simulink library "ddm"  (R2021b)
settings: Solver=VariableStepAuto  StartTime=0.0  StopTime=10.0  RelTol=1e-3
undefined symbols (not defined in the file or in its folder): ENUM_ADASACCSTA_ERROR, ENUM_ADASACCSTA_OFF, ENUM_ADASACCSTA_STANDBY, ENUM_ADASISASTA_OFF, ENUM_ALLOWMOV_ALLOWREADY, ENUM_APS, ENUM_BRKSTA_ERROR, ENUM_BRKSTA_OFF, ENUM_BRKSTA_ON, ENUM_CHGPREACTERRSTA_OBCPRE, ENUM_DCDCFAULTSTA_ANYFAULTLV1, ENUM_DCDCFAULTSTA_ANYFAULTLV2, ENUM_DRIVETRAIN_AWD, ENUM_DRIVETRAIN_FWD, ENUM_DRIVETRAIN_RWD, ENUM_DRSEATSTA_INVALID, ENUM_EDUDRTSTA_NORMAL, ENUM_EPBSTA_APPLIED, ENUM_EPBSTA_RELEASED, ENUM_HVBATTREADYPRE_READY, ENUM_MCUWARN_LV0, ENUM_MCUWARN_LV1, ENUM_MCUWARN_LV2, ENUM_MCUWARN_LV3, ENUM_MCUWARN_NOERROR, ENUM_OBCFAULTSTA_ANYFAULT, ENUM_PAS_R2F2, ENUM_PDFAULT_BATTPDFAIL, ENUM_PDFAULT_DCDCDISABLE, ENUM_PDFAULT_MCUDISABLE, ENUM_PDFAULT_MCUDISCHRG, ENUM_POWERSTA_OFF, ENUM_POWERSTA_ON, ENUM_POWERSTA_READY, ENUM_POWERSTA_STANDBY, ENUM_PRESSINDI_LOW, ENUM_PUFAULT_BATTUPFAIL, ENUM_PUFAULT_DCDCENABLEFAIL, ENUM_PUFAULT_PRECHRGCHKFAIL, ENUM_PUFAULT_SAFETYCHKFAIL, ENUM_PUSTATE_COMPLETED, ENUM_PWRSTASW_OFF, ENUM_PWRSTASW_OFFA, ENUM_PWRSTASW_OFFCHVCHRG, ENUM_PWRSTASW_OFFCLVCHRG, ENUM_PWRSTASW_ON, ENUM_PWRSTASW_ONHVCHRG, ENUM_PWRSTASW_READY, ENUM_PWRSTASW_STANDBY, ENUM_RANGESTA_12IN, ENUM_RANGESTA_12OUT, ENUM_SHIFTCOMMAND_D, ENUM_SHIFTCOMMAND_N, ENUM_SHIFTCOMMAND_P, ENUM_SHIFTCOMMAND_R, ENUM_ZONEMALFUNLV_1ST, ENUM_ZONEMALFUNLV_2ND, ENUM_ZONEMALFUNLV_3RD, ENUM_ZONEMALFUNLV_4TH, ENUM_ZONESPDCTRLMODE_ACC ... (+832)
libraries: hcu_lib x738, $bdroot x26, simulink x7
(part 15 of 25)

== system ddm/DDM/DDM/PMM/Comm err/VCU lost communication with CCU1 ==
  note: Fail Safe During Detection
  note: Test Pass Criteria
  note: Test Detection Criteria
  note: Fail Safe After Decision
  note: Release Condition After Failure Decision
  note: Release Condition During Failure Detection
  task_time_s : Inport
  VPMM_PowerSta_enum : Inport  Port=2
  VPMM_PwrStaSW_enum : Inport  Port=3
  VDDM_C3CCU1LCChk_flg : Inport  Port=4
  No_CAN3_BUS_OFF : Inport  Port=5
  DTC_clear_request : Inport  Port=6
  Constant15 : Constant  Value=KDDM_C3CCU1LCCFSSW_flg
  Constant{3,16,22,24} (4 alike) : Constant  Value=TRUE
  Constant18 : Constant  Value=KDDM_C3CCU1LCPassTO_s
  Constant19 : Constant  Value=KDDM_C3CCU1LCPassTO_s
  Constant{2,21,23,25,27} (5 alike) : Constant  Value=FALSE
  Constant20 : Constant  Value=KDDM_C3CCU1LCDFSSW_flg
  Constant26 : Constant  Value=ENUM_PWRSTASW_OFF
  Constant28 : Constant  Value=ENUM_PWRSTASW_OFF
  Constant4 : Constant  Value=ENUM_POWERSTA_OFF
  Constant40 : Constant  Value=KDDM_C3CCU1LCDTC_cnt
  Constant41 : Constant  Value=KDDM_C3CCU1LCDetTO_s
  Constant46 : Constant  Value=KDDM_C3CCU1LCDetSW_flg
  Constant48 : Constant  Value=KDDM_C3CCU1LCDTC_cnt
  Constant5 : Constant  Value=KDDM_C3CCU1LCPassSW_flg
  DTC_Couter : hcu_lib/Basic_Blocks/DTC_Couter
  DTC_Info : hcu_lib/Basic_Blocks/DTC_Info
  Data Type Conversion1 : DataTypeConversion  OutDataTypeStr=uint8
  Demux : Demux  Commented=on  Outputs=5
  Equal : RelationalOperator  Operator=~=  OutDataTypeStr=boolean  RndMeth=Simplest
  Equal2 : RelationalOperator  Operator=~=  OutDataTypeStr=boolean  RndMeth=Simplest
  Equal3 : RelationalOperator  OutDataTypeStr=boolean  RndMeth=Simplest
  Equal4 : RelationalOperator  Operator===  OutDataTypeStr=boolean  RndMeth=Simplest
  From19 : From  Commented=on  GotoTag=VDDM_C3CCU1LCDFS_flg
  Goto19 : Goto  Commented=on  GotoTag=VDDM_EDriveSysErrVCUErr_flg
  Logical Operator{2,5,12,15,18..19} (6 alike) : Logic  AllPortsSameDT=off  OutDataTypeStr=boolean
  Logical Operator21 : Logic  Operator=OR  AllPortsSameDT=off  OutDataTypeStr=boolean
  Logical Operator3 : Logic  Operator=OR  AllPortsSameDT=off  OutDataTypeStr=boolean
  Logical Operator6 : Logic  Operator=NOT  AllPortsSameDT=off  OutDataTypeStr=boolean
  Logical Operator8 : Logic  Operator=OR  AllPortsSameDT=off  OutDataTypeStr=boolean
  Relay : Relay  OnSwitchValue=ONE_INT  OffSwitchValue=ZERO_INT
  SR_Latch1 : Subsystem  mask(SR_Latch){}
      mask help: SR latch function.
  SR_Latch3 : hcu_lib/Basic_Blocks/SR_Latch
  SR_Latch4 : hcu_lib/Basic_Blocks/SR_Latch
  Switch{,1,4..7} (6 alike) : Switch  Criteria=u2 ~= 0
  Switch3 : Switch  Commented=on  Criteria=u2 ~= 0
  Test Detection Criteria : hcu_lib/Basic_Blocks/Test Detection Criteria
  Timer1 : hcu_lib/Basic_Blocks/Timer
  Unit Delay3 : UnitDelay  Commented=on  SampleTime=-1  HasFrameUpgradeWarning=on
  VDDM_C3CCU1LCDTC_raw32 : Outport
  VDDM_C3CCU1LCCFS_flg : Outport  Port=2
  wires:
  VPMM_PowerSta_enum/1 -> [VPMM_PowerSta_enum]
  VPMM_PwrStaSW_enum/1 -> [VPMM_PwrStaSW_enum]
  VDDM_C3CCU1LCChk_flg/1 -> [VDDM_C3CCU1LCChk_flg]
  task_time_s/1 -> [task_time_s]
  DTC_clear_request/1 -> [DTC_clear_request]
  No_CAN3_BUS_OFF/1 -> [No_CAN3_BUS_OFF]
  Equal4/1 -> Logical Operator8/1
  Switch4/1 -> [VDDM_C3CCU1LCCFSRls_flg]
  Constant20/1 -> Logical Operator12/1
  Constant25/1 -> Switch4/3
  [DTC_clear_request] -> Logical Operator8/2
  [VDDM_C3CCU1LCChk_flg] -> Switch6/1
  Equal3/1 -> SR_Latch1/1(set)
  Logical Operator8/1 -> Switch4/2
  SR_Latch1/1(latched) -> [VDDM_C3CCU1LCPass_flg]
  Switch7/1 -> [VDDM_C3CCU1LCDFSRls_flg]
  Constant46/1 -> Logical Operator19/2
  [VDDM_C3CCU1LCChk_flg] -> Switch5/1
  Constant23/1 -> Switch7/3
  From19/1 -> Switch3/2
  Test Detection Criteria/1 -> [VDDM_C3CCU1LCDet_flg]  "VDDM_C3CCU1LCDet_flg"
  Constant27/1 -> Switch5/3
  Switch6/1 -> Logical Operator6/1, Timer1/2
  Timer1/1 -> Equal3/1
  Constant16/1 -> Switch6/3
  Constant18/1 -> Timer1/4
  [VDDM_C3CCU1LCCFS_flg] -> Logical Operator21/2
  Equal2/1 -> Logical Operator5/2
  Switch/1 -> Goto19/1
  Constant26/1 -> Equal/2
  [VDDM_xxx_flg] -> SR_Latch1/2(reset)
  Data Type Conversion1/1 -> [VDDM_C3CCU1LCDTC_cnt]  "VDDM_C3CCU1LCDTC_cnt"
  Constant40/1 -> Test Detection Criteria/3
  [VDDM_C3CCU1LCCFSRls_flg] -> SR_Latch4/2
  DTC_Couter/1 -> SR_Latch4/1
  [No_CAN3_BUS_OFF] -> Logical Operator5/1
  Logical Operator18/1 -> [VDDM_C3CCU1LCCFS_flg]
  Logical Operator3/1 -> Logical Operator15/1
  [VDDM_C3CCU1LCPass_flg] -> Switch7/2
  Constant5/1 -> Logical Operator15/2
  Logical Operator2/1 -> Switch5/2
  Constant15/1 -> Logical Operator18/2
  Constant48/1 -> DTC_Couter/3
  Constant28/1 -> Equal2/2
  [VDDM_C3CCU1LCCFSRls_flg] -> Logical Operator3/2
  [VDDM_C3CCU1LCCFS_flg] -> Switch/2
  [No_CAN3_BUS_OFF] -> Logical Operator2/1
  [VDDM_C3CCU1LCPass_flg] -> Logical Operator3/1
  Logical Operator12/1 -> [VDDM_C3CCU1LCDFS_flg]
  Logical Operator21/1 -> SR_Latch3/2
  DTC_Couter/2 -> Data Type Conversion1/1
  Constant22/1 -> Switch7/1
  SR_Latch3/1 -> Logical Operator12/2
  Constant3/1 -> Switch/1
  Constant21/1 -> Switch/3
  Switch3/1 -> Demux/1
  [VDDM_C3CCU1LCDTC_cnt] -> Relay/1
  SR_Latch4/1 -> Logical Operator18/1
  Logical Operator5/1 -> Switch6/2
  Relay/1 -> SR_Latch3/1
  [VDDM_C3CCU1LCDFSRls_flg] -> Logical Operator21/1
  Constant4/1 -> Equal4/2
  [VDDM_C3CCU1LCDet_flg] -> Logical Operator19/1
  Logical Operator19/1 -> DTC_Couter/1
  Constant19/1 -> Equal3/2
  Logical Operator6/1 -> Timer1/1
  Equal/1 -> Logical Operator2/2
  [task_time_s] -> Test Detection Criteria/2
  Logical Operator15/1 -> DTC_Couter/2
  Demux/1 -> Unit Delay3/1
  Constant24/1 -> Switch4/1
  [VPMM_PowerSta_enum] -> Equal4/1
  [VPMM_PwrStaSW_enum] -> Equal/1
  [VPMM_PwrStaSW_enum] -> Equal2/1
  [task_time_s] -> Timer1/3
  DTC_Info/1 -> VDDM_C3CCU1LCDTC_raw32/1  "VDDM_C3CCU1LCDTC_raw32"
  [VDDM_C3CCU1LCPass_flg] -> DTC_Info/2
  [VDDM_C3CCU1LCCFS_flg] -> DTC_Info/3, VDDM_C3CCU1LCCFS_flg/1
  [VDDM_C3CCU1LCDet_flg] -> DTC_Info/1
  Constant41/1 -> Test Detection Criteria/4
  [DTC_clear_request] -> DTC_Info/4
  [DTC_clear_request] -> Switch1/2
  Switch1/1 -> Test Detection Criteria/1
  Switch5/1 -> [VDDM_xxx_flg], Switch1/3
  Constant2/1 -> Switch1/1

== system ddm/DDM/DDM/PMM/Comm err/VCU lost communication with CCU2 ==
  note: Fail Safe After Decision
  note: Test Pass Criteria
  note: Release Condition After Failure Decision
  note: Fail Safe During Detection
  note: Release Condition During Failure Detection
  note: Diagnostics and Fault Handling
  note: Test Detection Criteria
  task_time_s : Inport
  VPMM_PowerSta_enum : Inport  Port=2
  VPMM_PwrStaSW_enum : Inport  Port=3
  VDDM_C3CCU2LCChk_flg : Inport  Port=4
  No_CAN3_BUS_OFF : Inport  Port=5
  DTC_clear_request : Inport  Port=6
  Constant15 : Constant  Value=KDDM_C3CCU2LCCFSSW_flg
  Constant{3,16,22,24} (4 alike) : Constant  Value=TRUE
  Constant18 : Constant  Value=KDDM_C3CCU2LCPassTO_s
  Constant19 : Constant  Value=KDDM_C3CCU2LCPassTO_s
  Constant{2,21,23,25,27} (5 alike) : Constant  Value=FALSE
  Constant20 : Constant  Value=KDDM_C3CCU2LCDFSSW_flg
  Constant26 : Constant  Value=ENUM_PWRSTASW_OFF
  Constant28 : Constant  Value=ENUM_PWRSTASW_OFF
  Constant4 : Constant  Value=ENUM_POWERSTA_OFF
  Constant40 : Constant  Value=KDDM_C3CCU2LCDTC_cnt
  Constant41 : Constant  Value=KDDM_C3CCU2LCDetTO_s
  Constant46 : Constant  Value=KDDM_C3CCU2LCDetSW_flg
  Constant48 : Constant  Value=KDDM_C3CCU2LCDTC_cnt
  Constant5 : Constant  Value=KDDM_C3CCU2LCPassSW_flg
  DTC_Couter : hcu_lib/Basic_Blocks/DTC_Couter
  DTC_Info : hcu_lib/Basic_Blocks/DTC_Info
  Data Type Conversion1 : DataTypeConversion  OutDataTypeStr=uint8
  Demux : Demux  Commented=on  Outputs=5
  Equal : RelationalOperator  Operator=~=  OutDataTypeStr=boolean  RndMeth=Simplest
  Equal2 : RelationalOperator  Operator=~=  OutDataTypeStr=boolean  RndMeth=Simplest
  Equal3 : RelationalOperator  OutDataTypeStr=boolean  RndMeth=Simplest
  Equal4 : RelationalOperator  Operator===  OutDataTypeStr=boolean  RndMeth=Simplest
  From19 : From  Commented=on  GotoTag=VDDM_C3CCU2LCDFS_flg
  Goto19 : Goto  Commented=on  GotoTag=VDDM_EDriveSysErrVCUErr_flg
  Logical Operator{2,5,12,15,18..19} (6 alike) : Logic  AllPortsSameDT=off  OutDataTypeStr=boolean
  Logical Operator21 : Logic  Operator=OR  AllPortsSameDT=off  OutDataTypeStr=boolean
  Logical Operator3 : Logic  Operator=OR  AllPortsSameDT=off  OutDataTypeStr=boolean
  Logical Operator6 : Logic  Operator=NOT  AllPortsSameDT=off  OutDataTypeStr=boolean
  Logical Operator8 : Logic  Operator=OR  AllPortsSameDT=off  OutDataTypeStr=boolean
  Relay : Relay  OnSwitchValue=ONE_INT  OffSwitchValue=ZERO_INT
  SR_Latch1 : Subsystem  mask(SR_Latch){}
      mask help: SR latch function.
  SR_Latch3 : hcu_lib/Basic_Blocks/SR_Latch
  SR_Latch4 : hcu_lib/Basic_Blocks/SR_Latch
  Switch{,1,4..7} (6 alike) : Switch  Criteria=u2 ~= 0
  Switch3 : Switch  Commented=on  Criteria=u2 ~= 0
  Test Detection Criteria : hcu_lib/Basic_Blocks/Test Detection Criteria
  Timer1 : hcu_lib/Basic_Blocks/Timer
  Unit Delay3 : UnitDelay  Commented=on  SampleTime=-1  HasFrameUpgradeWarning=on
  VDDM_C3CCU2LCDTC_raw32 : Outport
  VDDM_C3CCU2LCCFS_flg : Outport  Port=2
  wires:
  task_time_s/1 -> [task_time_s]
  VDDM_C3CCU2LCChk_flg/1 -> [VDDM_C3CCU2LCChk_flg]
  VPMM_PwrStaSW_enum/1 -> [VPMM_PwrStaSW_enum]
  VPMM_PowerSta_enum/1 -> [VPMM_PowerSta_enum]
  No_CAN3_BUS_OFF/1 -> [No_CAN3_BUS_OFF]
  DTC_clear_request/1 -> [DTC_clear_request]
  Switch/1 -> Goto19/1
  Constant26/1 -> Equal/2
  Equal2/1 -> Logical Operator5/2
  [VDDM_C3CCU2LCCFS_flg] -> Logical Operator21/2
  Constant40/1 -> Test Detection Criteria/3
  Data Type Conversion1/1 -> [VDDM_C3CCU2LCDTC_cnt]  "VDDM_C3CCU2LCDTC_cnt"
  [VDDM_xxx_flg] -> SR_Latch1/2(reset)
  Logical Operator18/1 -> [VDDM_C3CCU2LCCFS_flg]
  [No_CAN3_BUS_OFF] -> Logical Operator5/1
  DTC_Couter/1 -> SR_Latch4/1
  Constant46/1 -> Logical Operator19/2
  SR_Latch1/1(latched) -> [VDDM_C3CCU2LCPass_flg]
  Constant23/1 -> Switch7/3
  Switch7/1 -> [VDDM_C3CCU2LCDFSRls_flg]
  Logical Operator8/1 -> Switch4/2
  Equal3/1 -> SR_Latch1/1(set)
  [VDDM_C3CCU2LCChk_flg] -> Switch6/1
  Constant20/1 -> Logical Operator12/1
  [DTC_clear_request] -> Logical Operator8/2
  Constant25/1 -> Switch4/3
  Equal4/1 -> Logical Operator8/1
  Switch4/1 -> [VDDM_C3CCU2LCCFSRls_flg]
  Constant3/1 -> Switch/1
  Constant22/1 -> Switch7/1
  [VDDM_C3CCU2LCChk_flg] -> Switch5/1
  DTC_Couter/2 -> Data Type Conversion1/1
  Constant48/1 -> DTC_Couter/3
  [VDDM_C3CCU2LCCFSRls_flg] -> Logical Operator3/2
  Logical Operator12/1 -> [VDDM_C3CCU2LCDFS_flg]
  Constant15/1 -> Logical Operator18/2
  Constant28/1 -> Equal2/2
  [VDDM_C3CCU2LCCFS_flg] -> Switch/2
  Equal/1 -> Logical Operator2/2
  Logical Operator6/1 -> Timer1/1
  Constant24/1 -> Switch4/1
  Constant19/1 -> Equal3/2
  [task_time_s] -> Test Detection Criteria/2
  [No_CAN3_BUS_OFF] -> Logical Operator2/1
  [VDDM_C3CCU2LCPass_flg] -> Logical Operator3/1
  Constant4/1 -> Equal4/2
  [VDDM_C3CCU2LCDFSRls_flg] -> Logical Operator21/1
  Relay/1 -> SR_Latch3/1
  Constant21/1 -> Switch/3
  [VDDM_C3CCU2LCDet_flg] -> Logical Operator19/1
  SR_Latch4/1 -> Logical Operator18/1
  Logical Operator21/1 -> SR_Latch3/2
  [VDDM_C3CCU2LCDTC_cnt] -> Relay/1
  Demux/1 -> Unit Delay3/1
  Switch3/1 -> Demux/1
  Logical Operator19/1 -> DTC_Couter/1
  Test Detection Criteria/1 -> [VDDM_C3CCU2LCDet_flg]  "VDDM_C3CCU2LCDet_flg"
  From19/1 -> Switch3/2
  Constant18/1 -> Timer1/4
  Constant16/1 -> Switch6/3
  [VDDM_C3CCU2LCCFSRls_flg] -> SR_Latch4/2
  Timer1/1 -> Equal3/1
  Switch6/1 -> Logical Operator6/1, Timer1/2
  Constant27/1 -> Switch5/3
  Logical Operator5/1 -> Switch6/2
  Constant5/1 -> Logical Operator15/2
  SR_Latch3/1 -> Logical Operator12/2
  [VDDM_C3CCU2LCPass_flg] -> Switch7/2
  Logical Operator3/1 -> Logical Operator15/1
  Logical Operator15/1 -> DTC_Couter/2
  Logical Operator2/1 -> Switch5/2
  [VPMM_PowerSta_enum] -> Equal4/1
  [VPMM_PwrStaSW_enum] -> Equal/1
  [VPMM_PwrStaSW_enum] -> Equal2/1
  [task_time_s] -> Timer1/3
  DTC_Info/1 -> VDDM_C3CCU2LCDTC_raw32/1  "VDDM_C3CCU2LCDTC_raw32"
  [VDDM_C3CCU2LCPass_flg] -> DTC_Info/2
  [VDDM_C3CCU2LCCFS_flg] -> DTC_Info/3, VDDM_C3CCU2LCCFS_flg/1
  [VDDM_C3CCU2LCDet_flg] -> DTC_Info/1
  Constant41/1 -> Test Detection Criteria/4
  [DTC_clear_request] -> DTC_Info/4
  [DTC_clear_request] -> Switch1/2
  Switch1/1 -> Test Detection Criteria/1
  Switch5/1 -> [VDDM_xxx_flg], Switch1/3
  Constant2/1 -> Switch1/1

== system ddm/DDM/DDM/PMM/Fault level/Fault level 1 subsystem error ==
  note: Fail Safe Operation During Failure Detection
  note: Release Condition During Failure Detection
  note: Fail Safe Operation After Failure Decision
  note: Test Pass Criteria
  note: Test Detection Criteria
  note: Diagnostics and Fault Handling
  note: Release Condition After Failure Decision
  task_time_s : Inport
  VPMM_PowerSta_enum : Inport  Port=2
  VPMM_PwrStaSW_enum : Inport  Port=3
  VDDM_C3BMS6LCCFS_flg : Inport  Port=4
  VDDM_C3CCU2LCCFS_flg : Inport  Port=5
  VDDM_MCUF1NoComCFS_flg : Inport  Port=6
  VDDM_MCUR1NoComCFS_flg : Inport  Port=7
  VINP_BMSWarn1_flg : Inport  Port=8
  VINP_BMSWarn2_flg : Inport  Port=9
  VINP_BMSWarn3_flg : Inport  Port=10
  VINP_DCDCFaultSta_enum : Inport  Port=11
  VINP_MCUWarnF_enum : Inport  Port=12
  VINP_MCUWarnR_enum : Inport  Port=13
  VINP_OBCFaultSta_enum : Inport  Port=14
  VPMM_DrivetrainSelect_enum : Inport  Port=15
  DTC_clear_request : Inport  Port=16
  No_CAN3_BUS_OFF : Inport  Port=17
  Constant : Constant  Value=KDDM_Lv1ErrDetTO_s
  Constant1 : Constant  Value=KDDM_Lv1ErrPassTO_s
  Constant{5,10,42,47} (4 alike) : Constant  Value=ENUM_MCUWARN_LV0
  Constant{6,11,43,49} (4 alike) : Constant  Value=ENUM_DRIVETRAIN_AWD
  Constant12 : Constant  Value=KDDM_Lv1ErrDTC_cnt
  Constant13 : Constant  Value=KDDM_Lv1ErrDetSW_flg
  Constant14 : Constant  Value=KDDM_Lv1ErrPassSW_flg
  Constant{15,21,25,27} (4 alike) : Constant  Value=FALSE
  Constant18 : Constant  Value=KDDM_Lv1ErrPassTO_s
  Constant2 : Constant  Value=KDDM_Lv1ErrCFSSW_flg
  Constant24 : Constant  Value=TRUE
  Constant26 : Constant  Value=ENUM_PWRSTASW_OFF
  Constant3 : Constant  Value=TRUE
  Constant36 : Constant  Value=ENUM_DCDCFAULTSTA_ANYFAULTLV1
  Constant37 : Constant  Value=ENUM_OBCFAULTSTA_ANYFAULT
  Constant38 : Constant  Value=ENUM_PWRSTASW_OFF
  Constant39 : Constant  Value=TRUE
  Constant4 : Constant  Value=ENUM_POWERSTA_OFF
  Constant40 : Constant  Value=KDDM_Lv1ErrDTC_cnt
  Constant44 : Constant  Value=ENUM_DRIVETRAIN_FWD
  Constant45 : Constant  Value=ENUM_DRIVETRAIN_RWD
  Constant50 : Constant  Value=ENUM_DCDCFAULTSTA_ANYFAULTLV1
  Constant51 : Constant  Value=ENUM_OBCFAULTSTA_ANYFAULT
  Constant7 : Constant  Value=ENUM_DRIVETRAIN_FWD
  Constant8 : Constant  Value=ENUM_DRIVETRAIN_RWD
  Constant9 : Constant  Value=KDDM_Lv1ErrDFSSW_flg
  DTC_Couter : hcu_lib/Basic_Blocks/DTC_Couter
  DTC_Info : hcu_lib/Basic_Blocks/DTC_Info
  Data Type Conversion1 : DataTypeConversion  OutDataTypeStr=uint8
  Equal : RelationalOperator  Operator=~=  OutDataTypeStr=boolean  RndMeth=Simplest
  Equal{1,4..9,14..21,25..26} (17 alike) : RelationalOperator  Operator===  OutDataTypeStr=boolean  RndMeth=Simplest
  Equal2 : RelationalOperator  Operator=~=  OutDataTypeStr=boolean  RndMeth=Simplest
  Equal3 : RelationalOperator  OutDataTypeStr=boolean  RndMeth=Simplest
  Goto24 : Goto  Commented=on  GotoTag=VDDM_EDriveSysErrVCUErr_flg
  Logical Operator{1,4..7,9..10,27..28} (9 alike) : Logic  Operator=NOT  AllPortsSameDT=off  OutDataTypeStr=boolean
  Logical Operator11 : Logic  Operator=OR  Inputs=7  AllPortsSameDT=off  OutDataTypeStr=boolean
  Logical Operator{12..13,15..16,18..19,22,24} (8 alike) : Logic  AllPortsSameDT=off  OutDataTypeStr=boolean
  Logical Operator{3,8,14,17,23,25} (6 alike) : Logic  Operator=OR  AllPortsSameDT=off  OutDataTypeStr=boolean
  Logical Operator2 : Logic  Inputs=6  AllPortsSameDT=off  OutDataTypeStr=boolean
  Logical Operator20 : Logic  Operator=OR  Inputs=7  AllPortsSameDT=off  OutDataTypeStr=boolean
  Logical Operator26 : Logic  Inputs=6  AllPortsSameDT=off  OutDataTypeStr=boolean
  Relay : Relay  OnSwitchValue=ONE_INT  OffSwitchValue=ZERO_INT
  SR_Latch1 : Subsystem  mask(SR_Latch){}
      mask help: SR latch function.
  SR_Latch3 : hcu_lib/Basic_Blocks/SR_Latch
  SR_Latch4 : hcu_lib/Basic_Blocks/SR_Latch
  Switch{,2,4..6} (5 alike) : Switch  Criteria=u2 ~= 0
  Test Detection Criteria : hcu_lib/Basic_Blocks/Test Detection Criteria
  Timer1 : hcu_lib/Basic_Blocks/Timer
  VDDM_Lv1ErrDTC_raw32 : Outport
  wires:
  task_time_s/1 -> [task_time_s]
  VPMM_PwrStaSW_enum/1 -> [VPMM_PwrStaSW_enum]
  VPMM_PowerSta_enum/1 -> [VPMM_PowerSta_enum]
  VDDM_C3CCU2LCCFS_flg/1 -> [VDDM_C3CCU2LCCFS_flg]
  VPMM_DrivetrainSelect_enum/1 -> [VPMM_DrivetrainSelect_enum]
  VINP_MCUWarnR_enum/1 -> [VINP_MCUWarnR_enum]
  VDDM_MCUR1NoComCFS_flg/1 -> [VDDM_MCUR1NoComCFS_flg]
  VDDM_MCUF1NoComCFS_flg/1 -> [VDDM_MCUF1NoComCFS_flg]
  VINP_BMSWarn1_flg/1 -> [VINP_BMSWarn1_flg]
  VINP_BMSWarn2_flg/1 -> [VINP_BMSWarn2_flg]
  VINP_BMSWarn3_flg/1 -> [VINP_BMSWarn3_flg]
  VINP_DCDCFaultSta_enum/1 -> [VINP_DCDCFaultSta_enum]
  VINP_MCUWarnF_enum/1 -> [VINP_MCUWarnF_enum]
  VINP_OBCFaultSta_enum/1 -> [VINP_OBCFaultSta_enum]
  VDDM_C3BMS6LCCFS_flg/1 -> [VDDM_C3BMS6LCCFS_flg]
  Equal4/1 -> Logical Operator8/1
  Constant1/1 -> Timer1/4
  Relay/1 -> SR_Latch3/1
  DTC_Couter/2 -> Data Type Conversion1/1
  Constant21/1 -> Switch/3
  Constant2/1 -> Logical Operator18/2
  Switch/1 -> Goto24/1
  [DTC_clear_request] -> Logical Operator8/2
  Constant3/1 -> Switch/1
  [VDDM_Lv1ErrDet_flg] -> Logical Operator19/1
  SR_Latch1/1(latched) -> [VDDM_Lv1ErrPass_flg]
  SR_Latch4/1 -> Logical Operator18/1
  Logical Operator18/1 -> [VDDM_Lv1ErrCFS_flg]
  Timer1/1 -> Equal3/1
  Constant25/1 -> Switch4/3
  Data Type Conversion1/1 -> [VDDM_Lv1ErrDTC_cnt]  "VDDM_Lv1ErrDTC_cnt"
  [VDDM_Lv1ErrCFSRls_flg] -> SR_Latch4/2
  Logical Operator1/1 -> Logical Operator2/3
  Equal3/1 -> SR_Latch1/1(set)
  Constant14/1 -> Logical Operator15/2
  [No_CAN3_BUS_OFF] -> Logical Operator2/1
  Constant12/1 -> DTC_Couter/3
  Logical Operator8/1 -> Switch4/2
  Logical Operator15/1 -> DTC_Couter/2
  Constant26/1 -> Equal/2
  Test Detection Criteria/1 -> [VDDM_Lv1ErrDet_flg]  "VDDM_Lv1ErrDet_flg"
  Constant27/1 -> Switch5/3
  Switch4/1 -> [VDDM_Lv1ErrCFSRls_flg]
  Constant9/1 -> Logical Operator12/1
  Logical Operator19/1 -> DTC_Couter/1
  [VDDM_C3BMS6LCCFS_flg] -> Logical Operator1/1
  Logical Operator2/1 -> Switch5/2
  [task_time_s] -> Test Detection Criteria/2
  [VDDM_Lv1ErrDTC_cnt] -> Relay/1
  Logical Operator12/1 -> [VDDM_Lv1ErrDFS_flg]
  Equal/1 -> Logical Operator2/2
  DTC_Couter/1 -> SR_Latch4/1
  SR_Latch3/1 -> Logical Operator12/2
  [VDDM_Lv1ErrPass_flg] -> Logical Operator3/1
  Constant40/1 -> Test Detection Criteria/3
  Constant24/1 -> Switch4/1
  Logical Operator6/1 -> Timer1/1
  [VDDM_Lv1ErrCFSRls_flg] -> Logical Operator3/2
  Constant18/1 -> Equal3/2
  Switch2/1 -> Logical Operator6/1, Timer1/2
  [VDDM_Lv1ErrCFS_flg] -> Switch/2
  Constant13/1 -> Logical Operator19/2
  Logical Operator3/1 -> Logical Operator15/1
  Constant4/1 -> Equal4/2
  Logical Operator7/1 -> Logical Operator2/4
  [VDDM_C3CCU2LCCFS_flg] -> Logical Operator7/1
  [VDDM_MCUF1NoComCFS_flg] -> Logical Operator9/1
  Logical Operator9/1 -> Logical Operator2/5
  [VDDM_MCUR1NoComCFS_flg] -> Logical Operator10/1
  Logical Operator10/1 -> Logical Operator2/6
  [VINP_BMSWarn2_flg] -> Logical Operator11/2
  [VINP_BMSWarn3_flg] -> Logical Operator11/3
  [VINP_DCDCFaultSta_enum] -> Equal14/1
  Constant36/1 -> Equal14/2
  [VINP_OBCFaultSta_enum] -> Equal15/1
  Constant37/1 -> Equal15/2
  Logical Operator11/1 -> Switch5/1
  [VINP_BMSWarn1_flg] -> Logical Operator11/1
  Equal14/1 -> Logical Operator11/6
  Equal15/1 -> Logical Operator11/7
  Equal25/1 -> Logical Operator22/1
  Logical Operator25/1 -> Logical Operator24/2
  Equal19/1 -> Logical Operator25/2
  Equal18/1 -> Logical Operator24/1
  Constant38/1 -> Equal2/2
  [No_CAN3_BUS_OFF] -> Logical Operator26/1
  Constant47/1 -> Equal18/2
  Logical Operator4/1 -> Logical Operator26/3
  [VDDM_C3BMS6LCCFS_flg] -> Logical Operator4/1
  [VINP_BMSWarn3_flg] -> Logical Operator20/3
  [VINP_BMSWarn1_flg] -> Logical Operator20/1
  [VINP_BMSWarn2_flg] -> Logical Operator20/2
  Logical Operator27/1 -> Logical Operator26/4
  Constant42/1 -> Equal25/2
  [VINP_DCDCFaultSta_enum] -> Equal20/1
  Equal26/1 -> Logical Operator23/2
  Logical Operator20/1 -> Switch2/1
  [VINP_OBCFaultSta_enum] -> Equal21/1
  Equal16/1 -> Logical Operator23/1
  Logical Operator26/1 -> Switch2/2
  Logical Operator23/1 -> Logical Operator22/2
  Equal21/1 -> Logical Operator20/7
  Equal20/1 -> Logical Operator20/6
  [VDDM_MCUR1NoComCFS_flg] -> Logical Operator5/1
  Equal2/1 -> Logical Operator26/2
  [VPMM_PwrStaSW_enum] -> Equal2/1
  Constant49/1 -> Equal19/2
  [VDDM_MCUF1NoComCFS_flg] -> Logical Operator28/1
  [VDDM_C3CCU2LCCFS_flg] -> Logical Operator27/1
  Constant50/1 -> Equal20/2
  Logical Operator5/1 -> Logical Operator26/6
  [VPMM_DrivetrainSelect_enum] -> Equal17/2, Equal19/1
  Logical Operator24/1 -> Logical Operator20/5
  Constant51/1 -> Equal21/2
  Constant39/1 -> Switch2/3
  Logical Operator22/1 -> Logical Operator20/4
  Constant43/1 -> Equal26/2
  Constant44/1 -> Equal16/1
  [VINP_MCUWarnF_enum] -> Equal25/1
  Constant45/1 -> Equal17/1
  [VINP_MCUWarnR_enum] -> Equal18/1
  [VPMM_DrivetrainSelect_enum] -> Equal16/2, Equal26/1
  Equal17/1 -> Logical Operator25/1
  Logical Operator28/1 -> Logical Operator26/5
  [VPMM_PowerSta_enum] -> Equal4/1
  [VPMM_PwrStaSW_enum] -> Equal/1
  Equal5/1 -> Logical Operator17/1
  [VPMM_DrivetrainSelect_enum] -> Equal9/1, Equal1/2
  [VINP_MCUWarnR_enum] -> Equal6/1
  Constant8/1 -> Equal5/1
  [VINP_MCUWarnF_enum] -> Equal8/1
  Constant7/1 -> Equal1/1
  Constant6/1 -> Equal9/2
  [VPMM_DrivetrainSelect_enum] -> Equal7/1, Equal5/2
  Constant11/1 -> Equal7/2
  Logical Operator14/1 -> Logical Operator13/2
  Equal1/1 -> Logical Operator14/1
  Equal9/1 -> Logical Operator14/2
  Constant5/1 -> Equal8/2
  Constant10/1 -> Equal6/2
  Equal6/1 -> Logical Operator16/1
  Equal7/1 -> Logical Operator17/2
  Logical Operator17/1 -> Logical Operator16/2
  Equal8/1 -> Logical Operator13/1
  Logical Operator13/1 -> Logical Operator11/4
  Logical Operator16/1 -> Logical Operator11/5
  DTC_clear_request/1 -> [DTC_clear_request]
  No_CAN3_BUS_OFF/1 -> [No_CAN3_BUS_OFF]
  [task_time_s] -> Timer1/3
  DTC_Info/1 -> VDDM_Lv1ErrDTC_raw32/1  "VDDM_Lv1ErrDTC_raw32"
  [VDDM_Lv1ErrPass_flg] -> DTC_Info/2
  [VDDM_Lv1ErrCFS_flg] -> DTC_Info/3
  [VDDM_Lv1ErrCFS_flg] -> SR_Latch3/2
  [VDDM_Lv1ErrDet_flg] -> DTC_Info/1
  Constant/1 -> Test Detection Criteria/4
  [DTC_clear_request] -> DTC_Info/4
  [DTC_clear_request] -> Switch6/2
  Switch6/1 -> Test Detection Criteria/1
  Switch5/1 -> [VDDM_xxx_flg], Switch6/3
  Constant15/1 -> Switch6/1
  [VDDM_xxx_flg] -> SR_Latch1/2(reset)

== system ddm/DDM/DDM/PMM/Fault level/Fault level 2 subsystem error ==
  note: Test Pass Criteria
  note: Release Condition During Failure Detection
  note: Fail Safe Operation During Failure Detection
  note: Test Detection Criteria
  note: Diagnostics and Fault Handling
  note: Fail Safe Operation After Failure Decision
  note: Release Condition After Failure Decision
  task_time_s : Inport
  VPMM_PowerSta_enum : Inport  Port=2
  VPMM_PwrStaSW_enum : Inport  Port=3
  VDDM_C3BMS6LCCFS_flg : Inport  Port=4
  VDDM_C3CCU2LCCFS_flg : Inport  Port=5
  VDDM_MCUF1NoComCFS_flg : Inport  Port=6
  VDDM_MCUR1NoComCFS_flg : Inport  Port=7
  VINP_BMSWarn4_flg : Inport  Port=8
  VINP_BMSWarn5_flg : Inport  Port=9
  VINP_DCDCFaultSta_enum : Inport  Port=10
  VINP_MCUWarnF_enum : Inport  Port=11
  VINP_MCUWarnR_enum : Inport  Port=12
  VPMM_DrivetrainSelect_enum : Inport  Port=13
  DTC_clear_request : Inport  Port=14
  No_CAN3_BUS_OFF : Inport  Port=15
  Constant1 : Constant  Value=ENUM_PWRSTASW_OFF
  Constant{6,10,30,34} (4 alike) : Constant  Value=ENUM_MCUWARN_LV2
  Constant{7,11,31,35} (4 alike) : Constant  Value=ENUM_DRIVETRAIN_AWD
  Constant12 : Constant  Value=ENUM_DCDCFAULTSTA_ANYFAULTLV2
  Constant{2,13,29,37} (4 alike) : Constant  Value=ENUM_MCUWARN_LV1
  Constant{14,21,25,27} (4 alike) : Constant  Value=FALSE
  Constant15 : Constant  Value=KDDM_Lv2ErrDetSW_flg
  Constant16 : Constant  Value=KDDM_Lv2ErrPassSW_flg
  Constant19 : Constant  Value=KDDM_Lv2ErrPassTO_s
  Constant20 : Constant  Value=KDDM_Lv2ErrCFSSW_flg
  Constant22 : Constant  Value=TRUE
  Constant23 : Constant  Value=ENUM_POWERSTA_OFF
  Constant24 : Constant  Value=TRUE
  Constant26 : Constant  Value=ENUM_PWRSTASW_OFF
  Constant3 : Constant  Value=KDDM_Lv2ErrDetTO_s
  Constant32 : Constant  Value=ENUM_DRIVETRAIN_FWD
  Constant33 : Constant  Value=ENUM_DRIVETRAIN_RWD
  Constant36 : Constant  Value=ENUM_DCDCFAULTSTA_ANYFAULTLV2
  Constant39 : Constant  Value=TRUE
  Constant4 : Constant  Value=KDDM_Lv2ErrPassTO_s
  Constant40 : Constant  Value=KDDM_Lv2ErrDTC_cnt
  Constant46 : Constant  Value=KDDM_Lv2ErrDFSSW_flg
  Constant5 : Constant  Value=KDDM_Lv2ErrDTC_cnt
  Constant8 : Constant  Value=ENUM_DRIVETRAIN_FWD
  Constant9 : Constant  Value=ENUM_DRIVETRAIN_RWD
  DTC_Couter : hcu_lib/Basic_Blocks/DTC_Couter
  DTC_Info : hcu_lib/Basic_Blocks/DTC_Info
  Data Type Conversion1 : DataTypeConversion  OutDataTypeStr=uint8
  Equal : RelationalOperator  Operator=~=  OutDataTypeStr=boolean  RndMeth=Simplest
  Equal1 : RelationalOperator  Operator=~=  OutDataTypeStr=boolean  RndMeth=Simplest
  Equal{2,4..21} (19 alike) : RelationalOperator  Operator===  OutDataTypeStr=boolean  RndMeth=Simplest
  Equal3 : RelationalOperator  OutDataTypeStr=boolean  RndMeth=Simplest
  Goto24 : Goto  Commented=on  GotoTag=VDDM_EDriveSysErrVCUErr_flg
  Logical Operator{1,4..7,9..10,31..32} (9 alike) : Logic  Operator=NOT  AllPortsSameDT=off  OutDataTypeStr=boolean
  Logical Operator11 : Logic  Operator=OR  Inputs=5  AllPortsSameDT=off  OutDataTypeStr=boolean
  Logical Operator{12..13,15..16,18..19,22,24} (8 alike) : Logic  AllPortsSameDT=off  OutDataTypeStr=boolean
  Logical Operator{3,8,14,17,23,25,27..30} (10 alike) : Logic  Operator=OR  AllPortsSameDT=off  OutDataTypeStr=boolean
  Logical Operator2 : Logic  Inputs=6  AllPortsSameDT=off  OutDataTypeStr=boolean
  Logical Operator20 : Logic  Operator=OR  Inputs=5  AllPortsSameDT=off  OutDataTypeStr=boolean
  Logical Operator26 : Logic  Inputs=6  AllPortsSameDT=off  OutDataTypeStr=boolean
  Relay : Relay  OnSwitchValue=ONE_INT  OffSwitchValue=ZERO_INT
  SR_Latch1 : Subsystem  mask(SR_Latch){}
      mask help: SR latch function.
  SR_Latch3 : hcu_lib/Basic_Blocks/SR_Latch
  SR_Latch4 : hcu_lib/Basic_Blocks/SR_Latch
  Switch{,2,4..6} (5 alike) : Switch  Criteria=u2 ~= 0
  Test Detection Criteria : hcu_lib/Basic_Blocks/Test Detection Criteria
  Timer1 : hcu_lib/Basic_Blocks/Timer
  VDDM_Lv2ErrDTC_raw32 : Outport
  wires:
  VINP_MCUWarnF_enum/1 -> [VINP_MCUWarnF_enum]
  VINP_DCDCFaultSta_enum/1 -> [VINP_DCDCFaultSta_enum]
  VDDM_MCUF1NoComCFS_flg/1 -> [VDDM_MCUF1NoComCFS_flg]
  VDDM_MCUR1NoComCFS_flg/1 -> [VDDM_MCUR1NoComCFS_flg]
  VINP_MCUWarnR_enum/1 -> [VINP_MCUWarnR_enum]
  VPMM_DrivetrainSelect_enum/1 -> [VPMM_DrivetrainSelect_enum]
  VDDM_C3CCU2LCCFS_flg/1 -> [VDDM_C3CCU2LCCFS_flg]
  VPMM_PowerSta_enum/1 -> [VPMM_PowerSta_enum]
  VPMM_PwrStaSW_enum/1 -> [VPMM_PwrStaSW_enum]
  task_time_s/1 -> [task_time_s]
  VINP_BMSWarn5_flg/1 -> [VINP_BMSWarn5_flg]
  VINP_BMSWarn4_flg/1 -> [VINP_BMSWarn4_flg]
  VDDM_C3BMS6LCCFS_flg/1 -> [VDDM_C3BMS6LCCFS_flg]
  Constant46/1 -> Logical Operator12/1
  Constant16/1 -> Logical Operator15/2
  Constant5/1 -> DTC_Couter/3
  Constant15/1 -> Logical Operator19/2
  [VDDM_Lv2ErrCFSRls_flg] -> Logical Operator3/2
  Equal9/1 -> Logical Operator14/2
  Equal10/1 -> Logical Operator14/1
  [VDDM_MCUF1NoComCFS_flg] -> Logical Operator9/1
  SR_Latch1/1(latched) -> [VDDM_Lv2ErrPass_flg]
  Constant39/1 -> Switch2/3
  Test Detection Criteria/1 -> [VDDM_Lv2ErrDet_flg]  "VDDM_Lv2ErrDet_flg"
  Constant21/1 -> Switch/3
  Logical Operator7/1 -> Logical Operator2/4
  [task_time_s] -> Test Detection Criteria/2
  [VINP_BMSWarn4_flg] -> Logical Operator11/1
  Logical Operator16/1 -> Logical Operator11/4
  [VINP_BMSWarn5_flg] -> Logical Operator11/2
  Logical Operator13/1 -> Logical Operator11/3
  Logical Operator6/1 -> Timer1/1
  Constant36/1 -> Equal14/2
  [No_CAN3_BUS_OFF] -> Logical Operator2/1
  [VPMM_DrivetrainSelect_enum] -> Equal13/1, Equal11/2
  Constant33/1 -> Equal11/1
  Constant31/1 -> Equal9/2
  Constant35/1 -> Equal13/2
  [VINP_MCUWarnR_enum] -> Equal12/1, Equal15/2
  Constant22/1 -> Switch/1
  Logical Operator12/1 -> [VDDM_Lv2ErrDFS_flg]
  Logical Operator17/1 -> Logical Operator16/2
  Logical Operator14/1 -> Logical Operator13/2
  Constant32/1 -> Equal10/1
  [VPMM_DrivetrainSelect_enum] -> Equal9/1, Equal10/2
  DTC_Couter/1 -> SR_Latch4/1
  Constant26/1 -> Equal/2
  Equal13/1 -> Logical Operator17/2
  Constant27/1 -> Switch5/3
  Constant30/1 -> Equal8/2
  [VDDM_C3CCU2LCCFS_flg] -> Logical Operator7/1
  Logical Operator10/1 -> Logical Operator2/6
  Logical Operator8/1 -> Switch4/2
  [VDDM_MCUR1NoComCFS_flg] -> Logical Operator10/1
  Logical Operator3/1 -> Logical Operator15/1
  Switch2/1 -> Timer1/2, Logical Operator6/1
  Logical Operator1/1 -> Logical Operator2/3
  Logical Operator9/1 -> Logical Operator2/5
  Logical Operator15/1 -> DTC_Couter/2
  SR_Latch3/1 -> Logical Operator12/2
  Constant24/1 -> Switch4/1
  Logical Operator19/1 -> DTC_Couter/1
  Logical Operator2/1 -> Switch5/2
  Constant19/1 -> Equal3/2
  Data Type Conversion1/1 -> [VDDM_Lv2ErrDTC_cnt]  "VDDM_Lv2ErrDTC_cnt"
  Timer1/1 -> Equal3/1
  [DTC_clear_request] -> Logical Operator8/2
  Equal4/1 -> Logical Operator8/1
  Logical Operator18/1 -> [VDDM_Lv2ErrCFS_flg]
  DTC_Couter/2 -> Data Type Conversion1/1
  Constant40/1 -> Test Detection Criteria/3
  Switch/1 -> Goto24/1
  Equal11/1 -> Logical Operator17/1
  [VDDM_C3BMS6LCCFS_flg] -> Logical Operator1/1
  [VDDM_Lv2ErrPass_flg] -> Logical Operator3/1
  Equal14/1 -> Logical Operator11/5
  Equal3/1 -> SR_Latch1/1(set)
  [VDDM_Lv2ErrCFS_flg] -> Switch/2
  Constant25/1 -> Switch4/3
  Equal/1 -> Logical Operator2/2
  [VDDM_Lv2ErrDet_flg] -> Logical Operator19/1
  Constant23/1 -> Equal4/2
  Constant34/1 -> Equal12/2
  [VINP_DCDCFaultSta_enum] -> Equal14/1
  Switch4/1 -> [VDDM_Lv2ErrCFSRls_flg]
  Logical Operator11/1 -> Switch5/1
  [VDDM_Lv2ErrDTC_cnt] -> Relay/1
  SR_Latch4/1 -> Logical Operator18/1
  Relay/1 -> SR_Latch3/1
  Constant20/1 -> Logical Operator18/2
  [VDDM_Lv2ErrCFSRls_flg] -> SR_Latch4/2
  [VINP_MCUWarnF_enum] -> Equal8/1, Equal7/2
  Constant4/1 -> Timer1/4
  Constant29/1 -> Equal7/1
  Equal7/1 -> Logical Operator29/1
  Equal8/1 -> Logical Operator29/2
  Logical Operator29/1 -> Logical Operator13/1
  Constant37/1 -> Equal15/1
  Equal15/1 -> Logical Operator30/1
  Equal12/1 -> Logical Operator30/2
  Logical Operator30/1 -> Logical Operator16/1
  [VPMM_PowerSta_enum] -> Equal4/1
  [VPMM_PwrStaSW_enum] -> Equal/1
  [VPMM_PwrStaSW_enum] -> Equal1/1
  Logical Operator28/1 -> Logical Operator24/1
  Equal6/1 -> Logical Operator28/2
  Equal18/1 -> Logical Operator28/1
  Constant13/1 -> Equal18/1
  Logical Operator27/1 -> Logical Operator22/1
  Equal20/1 -> Logical Operator27/2
  Equal19/1 -> Logical Operator27/1
  Constant2/1 -> Equal19/1
  [VINP_MCUWarnF_enum] -> Equal19/2, Equal20/1
  Logical Operator20/1 -> Switch2/1
  [VINP_DCDCFaultSta_enum] -> Equal17/1
  Constant10/1 -> Equal6/2
  Equal1/1 -> Logical Operator26/2
  Equal17/1 -> Logical Operator20/5
  [VDDM_C3BMS6LCCFS_flg] -> Logical Operator4/1
  Equal5/1 -> Logical Operator25/1
  Logical Operator26/1 -> Switch2/2
  Logical Operator32/1 -> Logical Operator26/5
  Logical Operator4/1 -> Logical Operator26/3
  [VDDM_MCUR1NoComCFS_flg] -> Logical Operator5/1
  Logical Operator5/1 -> Logical Operator26/6
  [VDDM_C3CCU2LCCFS_flg] -> Logical Operator31/1
  Constant6/1 -> Equal20/2
  Equal16/1 -> Logical Operator25/2
  Constant1/1 -> Equal1/2
  [VPMM_DrivetrainSelect_enum] -> Equal2/2, Equal21/1
  Constant8/1 -> Equal2/1
  Logical Operator23/1 -> Logical Operator22/2
  Logical Operator25/1 -> Logical Operator24/2
  [VINP_MCUWarnR_enum] -> Equal18/2, Equal6/1
  Constant11/1 -> Equal16/2
  Constant7/1 -> Equal21/2
  Constant9/1 -> Equal5/1
  [VPMM_DrivetrainSelect_enum] -> Equal5/2, Equal16/1
  [No_CAN3_BUS_OFF] -> Logical Operator26/1
  Constant12/1 -> Equal17/2
  Logical Operator22/1 -> Logical Operator20/3
  [VINP_BMSWarn5_flg] -> Logical Operator20/2
  Logical Operator24/1 -> Logical Operator20/4
  [VINP_BMSWarn4_flg] -> Logical Operator20/1
  Logical Operator31/1 -> Logical Operator26/4
  [VDDM_MCUF1NoComCFS_flg] -> Logical Operator32/1
  Equal2/1 -> Logical Operator23/1
  Equal21/1 -> Logical Operator23/2
  DTC_clear_request/1 -> [DTC_clear_request]
  No_CAN3_BUS_OFF/1 -> [No_CAN3_BUS_OFF]
  [task_time_s] -> Timer1/3
  DTC_Info/1 -> VDDM_Lv2ErrDTC_raw32/1  "VDDM_Lv2ErrDTC_raw32"
  [VDDM_Lv2ErrPass_flg] -> DTC_Info/2
  [VDDM_Lv2ErrCFS_flg] -> DTC_Info/3
  [VDDM_Lv2ErrCFS_flg] -> SR_Latch3/2
  [VDDM_Lv2ErrDet_flg] -> DTC_Info/1
  Constant3/1 -> Test Detection Criteria/4
  [DTC_clear_request] -> DTC_Info/4
  [DTC_clear_request] -> Switch6/2
  Switch6/1 -> Test Detection Criteria/1
  Switch5/1 -> [VDDM_xxx_flg], Switch6/3
  Constant14/1 -> Switch6/1
  [VDDM_xxx_flg] -> SR_Latch1/2(reset)

== system ddm/DDM/DDM/PMM/Fault level/Fault level 3 subsystem error ==
  note: Test Pass Criteria
  note: Release Condition During Failure Detection
  note: Fail Safe Operation During Failure Detection
  note: Test Detection Criteria
  note: Diagnostics and Fault Handling
  note: Fail Safe Operation After Failure Decision
  note: Release Condition After Failure Decision
  task_time_s : Inport
  VPMM_PowerSta_enum : Inport  Port=2
  VPMM_PwrStaSW_enum : Inport  Port=3
  VDDM_C3BMS6LCCFS_flg : Inport  Port=4
  VDDM_MCUF1NoComCFS_flg : Inport  Port=5
  VDDM_MCUR1NoComCFS_flg : Inport  Port=6
  VINP_BMSWarn6_flg : Inport  Port=7
  VINP_MCUWarnF_enum : Inport  Port=8
  VINP_MCUWarnR_enum : Inport  Port=9
  VPMM_DrivetrainSelect_enum : Inport  Port=10
  DTC_clear_request : Inport  Port=11
  No_CAN3_BUS_OFF : Inport  Port=12
  Constant{1,8,30,34} (4 alike) : Constant  Value=ENUM_MCUWARN_LV3
  Constant10 : Constant  Value=KDDM_Lv3ErrDetSW_flg
  Constant11 : Constant  Value=KDDM_Lv3ErrPassSW_flg
  Constant{12,21,25,27} (4 alike) : Constant  Value=FALSE
  Constant15 : Constant  Value=KDDM_Lv3ErrCFSSW_flg
  Constant16 : Constant  Value=TRUE
  Constant18 : Constant  Value=KDDM_Lv3ErrPassTO_s
  Constant19 : Constant  Value=ENUM_POWERSTA_OFF
  Constant{2,9,31,35} (4 alike) : Constant  Value=ENUM_DRIVETRAIN_AWD
  Constant20 : Constant  Value=KDDM_Lv3ErrDFSSW_flg
  Constant24 : Constant  Value=TRUE
  Constant26 : Constant  Value=ENUM_PWRSTASW_OFF
  Constant3 : Constant  Value=KDDM_Lv3ErrDetTO_s
  Constant32 : Constant  Value=ENUM_DRIVETRAIN_FWD
  Constant33 : Constant  Value=ENUM_DRIVETRAIN_RWD
  Constant38 : Constant  Value=ENUM_PWRSTASW_OFF
  Constant39 : Constant  Value=TRUE
  Constant4 : Constant  Value=KDDM_Lv3ErrPassTO_s
  Constant40 : Constant  Value=KDDM_Lv3ErrDTC_cnt
  Constant5 : Constant  Value=KDDM_Lv3ErrDTC_cnt
  Constant6 : Constant  Value=ENUM_DRIVETRAIN_FWD
  Constant7 : Constant  Value=ENUM_DRIVETRAIN_RWD
  DTC_Couter : hcu_lib/Basic_Blocks/DTC_Couter
  DTC_Info : hcu_lib/Basic_Blocks/DTC_Info
  Data Type Conversion1 : DataTypeConversion  OutDataTypeStr=uint8
  Equal : RelationalOperator  Operator=~=  OutDataTypeStr=boolean  RndMeth=Simplest
  Equal{1,4..15} (13 alike) : RelationalOperator  Operator===  OutDataTypeStr=boolean  RndMeth=Simplest
  Equal2 : RelationalOperator  Operator=~=  OutDataTypeStr=boolean  RndMeth=Simplest
  Equal3 : RelationalOperator  OutDataTypeStr=boolean  RndMeth=Simplest
  Goto24 : Goto  Commented=on  GotoTag=VDDM_EDriveSysErrVCUErr_flg
  Logical Operator{1,4..6,9..10,26} (7 alike) : Logic  Operator=NOT  AllPortsSameDT=off  OutDataTypeStr=boolean
  Logical Operator11 : Logic  Operator=OR  Inputs=3  AllPortsSameDT=off  OutDataTypeStr=boolean
  Logical Operator{12..13,15..16,18..20,23} (8 alike) : Logic  AllPortsSameDT=off  OutDataTypeStr=boolean
  Logical Operator{3,8,14,17,22,24} (6 alike) : Logic  Operator=OR  AllPortsSameDT=off  OutDataTypeStr=boolean
  Logical Operator2 : Logic  Inputs=5  AllPortsSameDT=off  OutDataTypeStr=boolean
  Logical Operator25 : Logic  Inputs=5  AllPortsSameDT=off  OutDataTypeStr=boolean
  Logical Operator7 : Logic  Operator=OR  Inputs=3  AllPortsSameDT=off  OutDataTypeStr=boolean
  Relay : Relay  OnSwitchValue=ONE_INT  OffSwitchValue=ZERO_INT
  SR_Latch1 : Subsystem  mask(SR_Latch){}
      mask help: SR latch function.
  SR_Latch3 : hcu_lib/Basic_Blocks/SR_Latch
  SR_Latch4 : hcu_lib/Basic_Blocks/SR_Latch
  Switch{,2,4..6} (5 alike) : Switch  Criteria=u2 ~= 0
  Test Detection Criteria : hcu_lib/Basic_Blocks/Test Detection Criteria
  Timer1 : hcu_lib/Basic_Blocks/Timer
  VDDM_Lv3ErrDTC_raw32 : Outport
  wires:
  VINP_BMSWarn6_flg/1 -> [VINP_BMSWarn6_flg]
  task_time_s/1 -> [task_time_s]
  VPMM_PwrStaSW_enum/1 -> [VPMM_PwrStaSW_enum]
  VPMM_PowerSta_enum/1 -> [VPMM_PowerSta_enum]
  VPMM_DrivetrainSelect_enum/1 -> [VPMM_DrivetrainSelect_enum]
  VINP_MCUWarnR_enum/1 -> [VINP_MCUWarnR_enum]
  VDDM_MCUR1NoComCFS_flg/1 -> [VDDM_MCUR1NoComCFS_flg]
  VDDM_MCUF1NoComCFS_flg/1 -> [VDDM_MCUF1NoComCFS_flg]
  VINP_MCUWarnF_enum/1 -> [VINP_MCUWarnF_enum]
  VDDM_C3BMS6LCCFS_flg/1 -> [VDDM_C3BMS6LCCFS_flg]
  [VINP_BMSWarn6_flg] -> Logical Operator11/1
  Constant20/1 -> Logical Operator12/1
  Constant11/1 -> Logical Operator15/2
  Constant5/1 -> DTC_Couter/3
  Constant10/1 -> Logical Operator19/2
  [VDDM_Lv3ErrCFSRls_flg] -> Logical Operator3/2
  Equal9/1 -> Logical Operator14/2
  Equal10/1 -> Logical Operator14/1
  [VDDM_MCUF1NoComCFS_flg] -> Logical Operator9/1
  SR_Latch1/1(latched) -> [VDDM_Lv3ErrPass_flg]
  Constant39/1 -> Switch2/3
  Test Detection Criteria/1 -> [VDDM_Lv3ErrDet_flg]  "VDDM_Lv3ErrDet_flg"
  Constant21/1 -> Switch/3
  [task_time_s] -> Test Detection Criteria/2
  Logical Operator16/1 -> Logical Operator11/3
  Logical Operator13/1 -> Logical Operator11/2
  Logical Operator6/1 -> Timer1/1
  [No_CAN3_BUS_OFF] -> Logical Operator2/1
  [VPMM_DrivetrainSelect_enum] -> Equal11/2, Equal13/1
  Constant33/1 -> Equal11/1
  Constant31/1 -> Equal9/2
  Constant35/1 -> Equal13/2
  [VINP_MCUWarnR_enum] -> Equal12/1
  Constant16/1 -> Switch/1
  Logical Operator12/1 -> [VDDM_Lv3ErrDFS_flg]
  Logical Operator17/1 -> Logical Operator16/2
  Logical Operator14/1 -> Logical Operator13/2
  Constant32/1 -> Equal10/1
  Equal12/1 -> Logical Operator16/1
  [VPMM_DrivetrainSelect_enum] -> Equal10/2, Equal9/1
  DTC_Couter/1 -> SR_Latch4/1
  Equal8/1 -> Logical Operator13/1
  Constant30/1 -> Equal8/2
  Logical Operator10/1 -> Logical Operator2/5
  Logical Operator8/1 -> Switch4/2
  [VDDM_MCUR1NoComCFS_flg] -> Logical Operator10/1
  Logical Operator3/1 -> Logical Operator15/1
  Constant27/1 -> Switch5/3
  Switch2/1 -> Logical Operator6/1, Timer1/2
  Logical Operator1/1 -> Logical Operator2/3
  Logical Operator9/1 -> Logical Operator2/4
  Logical Operator15/1 -> DTC_Couter/2
  SR_Latch3/1 -> Logical Operator12/2
  Constant24/1 -> Switch4/1
  Logical Operator19/1 -> DTC_Couter/1
  Equal13/1 -> Logical Operator17/2
  Logical Operator2/1 -> Switch5/2
  Constant18/1 -> Equal3/2
  Data Type Conversion1/1 -> [VDDM_Lv3ErrDTC_cnt]  "VDDM_Lv3ErrDTC_cnt"
  Constant26/1 -> Equal/2
  Timer1/1 -> Equal3/1
  [DTC_clear_request] -> Logical Operator8/2
  Equal4/1 -> Logical Operator8/1
  Logical Operator18/1 -> [VDDM_Lv3ErrCFS_flg]
  DTC_Couter/2 -> Data Type Conversion1/1
  Constant40/1 -> Test Detection Criteria/3
  Switch/1 -> Goto24/1
  Equal11/1 -> Logical Operator17/1
  [VDDM_C3BMS6LCCFS_flg] -> Logical Operator1/1
  [VDDM_Lv3ErrPass_flg] -> Logical Operator3/1
  Equal3/1 -> SR_Latch1/1(set)
  [VDDM_Lv3ErrCFS_flg] -> Switch/2
  Constant25/1 -> Switch4/3
  Equal/1 -> Logical Operator2/2
  Constant34/1 -> Equal12/2
  [VDDM_Lv3ErrDet_flg] -> Logical Operator19/1
  Constant19/1 -> Equal4/2
  Switch4/1 -> [VDDM_Lv3ErrCFSRls_flg]
  Logical Operator11/1 -> Switch5/1
  [VDDM_Lv3ErrDTC_cnt] -> Relay/1
  SR_Latch4/1 -> Logical Operator18/1
  Relay/1 -> SR_Latch3/1
  Constant15/1 -> Logical Operator18/2
  [VDDM_Lv3ErrCFSRls_flg] -> SR_Latch4/2
  [VINP_MCUWarnF_enum] -> Equal8/1
  Constant4/1 -> Timer1/4
  [VINP_BMSWarn6_flg] -> Logical Operator7/1
  Logical Operator7/1 -> Switch2/1
  [VDDM_MCUF1NoComCFS_flg] -> Logical Operator26/1
  [No_CAN3_BUS_OFF] -> Logical Operator25/1
  [VDDM_C3BMS6LCCFS_flg] -> Logical Operator4/1
  Constant38/1 -> Equal2/2
  [VDDM_MCUR1NoComCFS_flg] -> Logical Operator5/1
  Logical Operator4/1 -> Logical Operator25/3
  Logical Operator5/1 -> Logical Operator25/5
  Equal2/1 -> Logical Operator25/2
  Logical Operator26/1 -> Logical Operator25/4
  Logical Operator25/1 -> Switch2/2
  [VPMM_PowerSta_enum] -> Equal4/1
  [VPMM_PwrStaSW_enum] -> Equal/1
  [VPMM_PwrStaSW_enum] -> Equal2/1
  [VINP_MCUWarnF_enum] -> Equal14/1
  Constant8/1 -> Equal6/2
  Equal5/1 -> Logical Operator24/1
  Equal7/1 -> Logical Operator24/2
  Constant1/1 -> Equal14/2
  Equal14/1 -> Logical Operator20/1
  [VPMM_DrivetrainSelect_enum] -> Equal15/1, Equal1/2
  Equal6/1 -> Logical Operator23/1
  Constant6/1 -> Equal1/1
  Logical Operator22/1 -> Logical Operator20/2
  Logical Operator24/1 -> Logical Operator23/2
  [VINP_MCUWarnR_enum] -> Equal6/1
  Constant9/1 -> Equal7/2
  Constant2/1 -> Equal15/2
  Constant7/1 -> Equal5/1
  [VPMM_DrivetrainSelect_enum] -> Equal7/1, Equal5/2
  Equal1/1 -> Logical Operator22/1
  Equal15/1 -> Logical Operator22/2
  Logical Operator23/1 -> Logical Operator7/3
  Logical Operator20/1 -> Logical Operator7/2
  DTC_clear_request/1 -> [DTC_clear_request]
  No_CAN3_BUS_OFF/1 -> [No_CAN3_BUS_OFF]
  [task_time_s] -> Timer1/3
  DTC_Info/1 -> VDDM_Lv3ErrDTC_raw32/1  "VDDM_Lv3ErrDTC_raw32"
  [VDDM_Lv3ErrPass_flg] -> DTC_Info/2
  [VDDM_Lv3ErrCFS_flg] -> DTC_Info/3
  [VDDM_Lv3ErrCFS_flg] -> SR_Latch3/2
  [VDDM_Lv3ErrDet_flg] -> DTC_Info/1
  Constant3/1 -> Test Detection Criteria/4
  [DTC_clear_request] -> DTC_Info/4
  [DTC_clear_request] -> Switch6/2
  Switch6/1 -> Test Detection Criteria/1
  Switch5/1 -> [VDDM_xxx_flg], Switch6/3
  Constant12/1 -> Switch6/1
  [VDDM_xxx_flg] -> SR_Latch1/2(reset)
